simulink model "OutputToVisualizationTimeDet"  (R2016b)
settings: Solver=FixedStepDiscrete  StartTime=0.0  StopTime=10.0  FixedStep=sCoreParams.core.stepPeriod  RelTol=1e-3  EnableMultiTasking=on
undefined symbols (not defined in the file or in its folder): sCoreParams, sCoreParams_viz_featureInds
libraries: slrtlib x2, xpcrtudplib x2, xpcutilitieslib x1, xpcobsoletelib x1
settings Model: DataTypeOverride=Double  MinMaxOverflowLogging=ForceOff  Creator=rzelmann  LastModifiedBy=rzelmann
settings SolverCC: EnableConcurrentExecution=on  ConcurrentTasks=on  AutoInsertRateTranBlk=on
settings DataIOCC: SaveFormat=StructureWithTime  SaveOutput=off  SignalLogging=off  DSMLogging=off  SaveTime=off
settings OptimizationCC: BlockReduction=off  DefaultParameterBehavior=Inlined  LifeSpan=inf
settings DebuggingCC: AllowSymbolicDim=off  SFUnexpectedBacktrackingDiag=warning  SFNoUnconditionalDefaultTransitionDiag=warning  SFExecutionAtInitializationDiag=none
settings HardwareCC: ProdBitPerPointer=32  ProdBitPerSizeT=32  ProdBitPerPtrDiffT=32  ProdLargestAtomicFloat=None  ProdWordSize=32  ProdLongLongMode=on  ProdHWDeviceType=Generic->32-bit x86 compatible
settings ModelReferenceCC: UpdateModelReferenceTargets=Force  ParallelModelReferenceMATLABWorkerInit=Load Top Model  ModelReferenceNumInstancesAllowed=Single  ModelReferencePassRootInputsByReference=off
settings RTWCC: SystemTargetFile=slrt.tlc  TemplateMakefile=slrt_default_tmf  Description=Simulink Real-Time  RTWCompilerOptimization=on
settings CodeAppCC: MaxIdLength=63
settings ConfigComp: CovMetricSettings=dw  CovHtmlReporting=on  CovSaveCumulativeToWorkspaceVar=on  CovSaveSingleToWorkspaceVar=on  CovExternalEMLEnable=off

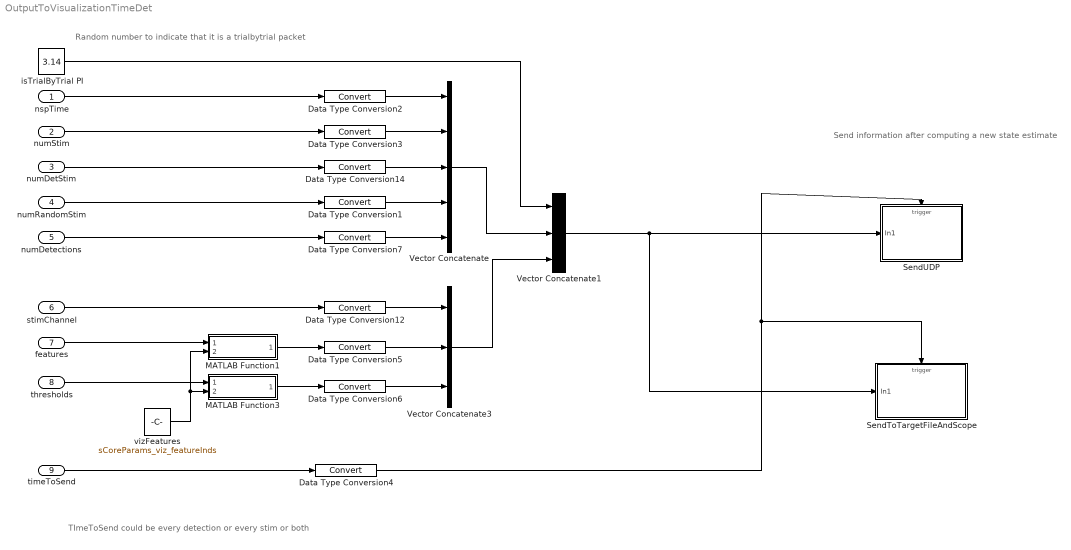
== system OutputToVisualizationTimeDet ==
  note: TImeToSend could be every detection or every stim or both
  note: Random number to indicate that it is a trialbytrial packet
  note: Send information after computing a new state estimate
  nspTime : Inport  SampleTime=sCoreParams.core.stepPeriod
  numStim : Inport  Port=2  OutDataTypeStr=double  SampleTime=sCoreParams.core.stepPeriod
  numDetStim : Inport  Port=3  OutDataTypeStr=double  SampleTime=sCoreParams.core.stepPeriod
  numRandomStim : Inport  Port=4  SampleTime=sCoreParams.core.stepPeriod
  numDetections : Inport  Port=5  SampleTime=sCoreParams.core.stepPeriod
  stimChannel : Inport  Port=6  OutDataTypeStr=int32  PortDimensions=[1 2]  SampleTime=sCoreParams.core.stepPeriod  Interpolate=off
  features : Inport  Port=7  PortDimensions=[1 sCoreParams.decoders.txDetector.nFeaturesUsedInDetection]  SampleTime=sCoreParams.core.stepPeriod
  thresholds : Inport  Port=8  PortDimensions=[1 sCoreParams.decoders.txDetector.nFeaturesUsedInDetection]  SampleTime=sCoreParams.core.stepPeriod
  timeToSend : Inport  Port=9  OutDataTypeStr=boolean  PortDimensions=1  SampleTime=sCoreParams.core.stepPeriod
  Data Type Conversion{1..7,12,14} (9 alike) : DataTypeConversion
  MATLAB Function1 : MATLAB Function  TreatAsAtomicUnit=on
  MATLAB Function3 : MATLAB Function  TreatAsAtomicUnit=on
  SendToTargetFileAndScope : Subsystem
  SendUDP : Subsystem
  Vector Concatenate : Concatenate  NumInputs=5
  Vector Concatenate1 : Concatenate  NumInputs=3
  Vector Concatenate3 : Concatenate  NumInputs=3
  isTrialByTrial PI : Constant  Value=3.14
  vizFeatures : Constant  Value=sCoreParams_viz_featureInds
  wires:
  thresholds/1 -> MATLAB Function3/1(signalIn)
  Data Type Conversion2/1 -> Vector Concatenate/1
  MATLAB Function3/1(signalOut) -> Data Type Conversion6/1
  Vector Concatenate/1 -> Vector Concatenate1/2
  Vector Concatenate3/1 -> Vector Concatenate1/3
  Vector Concatenate1/1 -> SendToTargetFileAndScope/1(In1), SendUDP/1(In1)
  stimChannel/1 -> Data Type Conversion12/1
  nspTime/1 -> Data Type Conversion2/1
  numStim/1 -> Data Type Conversion3/1
  features/1 -> MATLAB Function1/1(signalIn)
  numRandomStim/1 -> Data Type Conversion1/1
  Data Type Conversion5/1 -> Vector Concatenate3/2
  numDetStim/1 -> Data Type Conversion14/1
  Data Type Conversion14/1 -> Vector Concatenate/3
  timeToSend/1 -> Data Type Conversion4/1
  Data Type Conversion3/1 -> Vector Concatenate/2
  Data Type Conversion1/1 -> Vector Concatenate/4
  Data Type Conversion12/1 -> Vector Concatenate3/1
  isTrialByTrial PI/1 -> Vector Concatenate1/1
  Data Type Conversion4/1 -> SendToTargetFileAndScope/Trigger, SendUDP/Trigger
  Data Type Conversion6/1 -> Vector Concatenate3/3
  numDetections/1 -> Data Type Conversion7/1
  Data Type Conversion7/1 -> Vector Concatenate/5
  vizFeatures/1 -> MATLAB Function1/2(selectCh), MATLAB Function3/2(selectCh)
  MATLAB Function1/1(signalOut) -> Data Type Conversion5/1

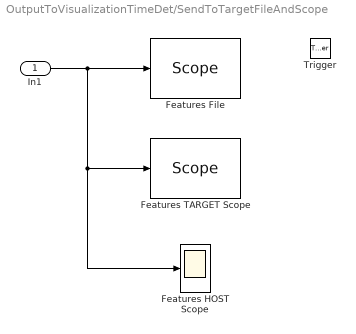
== system OutputToVisualizationTimeDet/SendToTargetFileAndScope ==
  In1 : Inport
  Trigger : TriggerPort  VariantControl=Variant  PortDimensions=1
  Features File : slrtlib/Displays and Logging/Scope   scopeno=2  scopetype=File  autostart=on  viewmode=Graphical redraw  formatstr='%15.6f'  grid=on  ylimits=[0,0]  nosamples=1000  noprepostsamples=-10  interleave=1  triggermode=FreeRun  triggersignal=1  trigsignalfromport=on  triggerlevel=0.0  triggerslope=Rising  triggerscope=1  triggersample=0  filename=feat_<%%%>.dat  mode=Lazy  writesize=512  autorestart=on  dynamicfilemode=on  maxwritefilesize=512*1024^2
  Features HOST Scope : Scope
  Features TARGET Scope : slrtlib/Displays and Logging/Scope   scopeno=3  scopetype=Target  autostart=on  viewmode=Graphical sliding  formatstr='%15.6f'  grid=on  ylimits=[0,0]  nosamples=1000  noprepostsamples=0  interleave=1  triggermode=FreeRun  triggersignal=1  trigsignalfromport=on  triggerlevel=0.0  triggerslope=Rising  triggerscope=1  triggersample=0  filename=data.dat  mode=Lazy  writesize=512  autorestart=off  dynamicfilemode=off  maxwritefilesize=512*1024^2
  wires:
  In1/1 -> Features HOST Scope/1, Features TARGET Scope/1, Features File/1

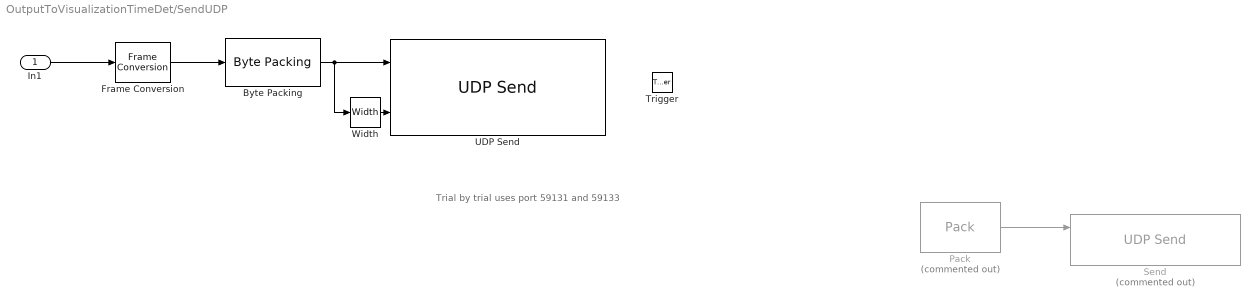
== system OutputToVisualizationTimeDet/SendUDP ==
  note: Trial by trial uses port 59131 and 59133
  In1 : Inport
  Trigger : TriggerPort  VariantControl=Variant  PortDimensions=1
  "Byte Packing " : xpcutilitieslib/Byte Packing   MaskPackedDataType=uint8  MaskUnpackedDataTypes={'double'}  MaskAlignment=1
  Frame Conversion : FrameConversion  InheritSamplingMode=off  OutFrame=Sample-based
  Pack : xpcobsoletelib/Utilities/Pack   Commented=on  datatypes={'double'}  byteAlign=1
  Send : xpcrtudplib/UDP Send  Commented=on  ipAddressVal=Use host-target connection  localPort=59121  toAddress=255.255.255.255  toPort=59123  sampleTime=-1
  UDP Send : xpcrtudplib/UDP Send  ipAddressVal=Use host-target connection  localPort=59131  toAddress=255.255.255.255  toPort=59133  sampleTime=-1
  Width : Width
  wires:
  "Byte Packing "/1 -> Width/1, UDP Send/1
  In1/1 -> Frame Conversion/1
  Frame Conversion/1 -> "Byte Packing "/1
  Pack/1 -> Send/1
  Width/1 -> UDP Send/2

== matlab function OutputToVisualizationTimeDet/MATLAB Function1 ==
  data: signalIn input; signalOut output size=[1 length(sCoreParams_viz_featureInds)]; selectCh input
function signalOut = selectChannels(signalIn,selectCh)
%#codegen
signalOut = signalIn(:,selectCh);
%signalOut = selectChannels_EML(signalIn,selectCh);

== matlab function OutputToVisualizationTimeDet/MATLAB Function3 ==
  data: signalIn input; signalOut output size=[1 length(sCoreParams_viz_featureInds)]; selectCh input
function signalOut = selectChannels(signalIn,selectCh)
%#codegen
signalOut = signalIn(:,selectCh);
%signalOut = selectChannels_EML(signalIn,selectCh);
